simulink model "MPPT_vcte_temp"  (Simulink 7.4)
settings: Solver=ode3  StartTime=0.0  StopTime=6  FixedStep=1e-3  RelTol=1e-3
InitFcn:
  | % Ponto de linearização
  | D = 0.5;
  | L = 0.1;
  | C = 0.01;
  | R = 10;
  | Vo = 24;
  | Leq = L/(1-D)^2;
  | N = 1/(1-D);
libraries: simulink x4, powerlib_extras x1
settings Model: Creator=Luigi2  LastModifiedBy=Batlab
settings OptimizationCC: InitFltsAndDblsToZero=on
settings DebuggingCC: SaveWithParameterizedLinksMsg=none
settings GRTTargetCC: TargetFcnLib=ansi_tfl_tmw.mat

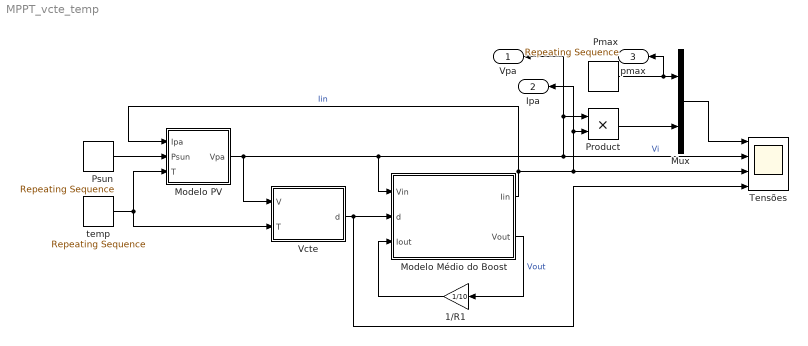
== system MPPT_vcte_temp ==
  1/R1 : Gain  Gain=1/10  ParameterDataType=sfix(16)  ParameterScaling=2^0  OutDataType=sfix(16)  OutScaling=2^0
  Modelo Médio do Boost : Subsystem  mask(Modelo de Pequenos Sinais do Boost){L=0.1, Iini=0, C=0.01, Vini=24}
      mask prompts: L "Indutância"; Iini "Corrente inicial"; C "Capacitância"; Vini "Tensão inicial"
      mask help:
      | São entradas do bloco:
      | Vin: Tensão de entrada
      | Iout: Corrente de saída
      | d: ciclo de trabalho
      |
      | São saídas do bloco:
      | Vout: Tensão de saída
      | Iin: Corrente de entrada
      |
      | Devem ser especificados a indutância, a capacitância e os seus valores iniciais para a utilização do modelo.
  Modelo PV : Subsystem
  Mux : Mux  Inputs=2
  Pmax : simulink/Sources/Repeating Sequence  SystemSampleTime=-1  rep_seq_t=[0 2 2 4 4 6]  rep_seq_y=[98.6721 98.6721 187.4175 187.4175 98.6721 98.6721]
  Product : Product  OutDataType=sfix(16)  OutScaling=2^0  RndMeth=Zero
  Psun : simulink/Sources/Repeating Sequence  SystemSampleTime=-1  rep_seq_t=[0 2 2 4 4 6]  rep_seq_y=[500 500 1000 1000 500 500]
  Tensões : Scope  NumInputPorts=4
      settings: TimeRange=6  YMin=-50~0~-2~0  YMax=250~40~10~0.4
  Vcte : Subsystem
  temp : simulink/Sources/Repeating Sequence  SystemSampleTime=-1  rep_seq_t=[0 2 2 4 4 6]  rep_seq_y=[25 25 40 40 25 25]
  Vpa : Outport  OutDataType=sfix(16)  OutScaling=2^0
  Ipa : Outport  Port=2  OutDataType=sfix(16)  OutScaling=2^0
  pmax : Outport  Port=3  OutDataType=sfix(16)  OutScaling=2^0
  wires:
  Modelo PV/1(Vpa) -> Tensões/2, Product/1, Vpa/1, Modelo Médio do Boost/1(Vin), Vcte/1(V)  "Vi"
  Modelo Médio do Boost/2(Vout) -> 1/R1/1  "Vout"
  1/R1/1 -> Modelo Médio do Boost/3(Iout)
  Modelo Médio do Boost/1(Iin) -> Tensões/3, Product/2, Ipa/1, Modelo PV/1(Ipa)  "Iin"
  Vcte/1(d) -> Tensões/4, Modelo Médio do Boost/2(d)
  Product/1 -> Mux/2
  Psun/1 -> Modelo PV/2(Psun)
  Pmax/1 -> Mux/1, pmax/1
  Mux/1 -> Tensões/1
  temp/1 -> Modelo PV/3(T), Vcte/2(T)

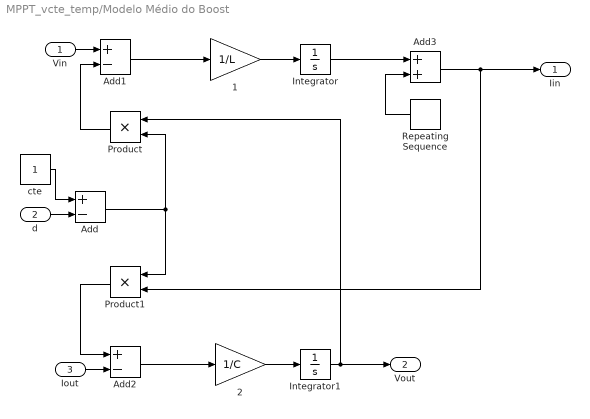
== system MPPT_vcte_temp/Modelo Médio do Boost ==
  Vin : Inport  OutDataType=sfix(16)  OutScaling=2^0
  d : Inport  Port=2  OutDataType=sfix(16)  OutScaling=2^0
  Iout : Inport  Port=3  OutDataType=sfix(16)  OutScaling=2^0
  1 : Gain  Gain=1/L  ParameterDataType=sfix(16)  ParameterScaling=2^0  OutDataType=sfix(16)  OutScaling=2^0
  2 : Gain  Gain=1/C  ParameterDataType=sfix(16)  ParameterScaling=2^0  OutDataType=sfix(16)  OutScaling=2^0
  Add : Sum  Inputs=+-  OutDataType=sfix(16)  OutScaling=2^-10
  Add1 : Sum  Inputs=+-  OutDataType=sfix(16)  OutScaling=2^-10
  Add2 : Sum  Inputs=+-  OutDataType=sfix(16)  OutScaling=2^-10
  Add3 : Sum  OutDataType=sfix(16)  OutScaling=2^-10
  Integrator : Integrator  InitialCondition=Iini
  Integrator1 : Integrator  InitialCondition=Vini
  Product : Product  OutDataType=sfix(16)  OutScaling=2^0  RndMeth=Zero
  Product1 : Product  OutDataType=sfix(16)  OutScaling=2^0  RndMeth=Zero
  Repeating Sequence : simulink/Sources/Repeating Sequence  SystemSampleTime=-1  rep_seq_t=[0 0.5/100 1/100]  rep_seq_y=[-1 1 -1]
  cte : Constant  OutDataType=sfix(16)  OutScaling=2^0
  Iin : Outport  OutDataType=sfix(16)  OutScaling=2^0
  Vout : Outport  Port=2  OutDataType=sfix(16)  OutScaling=2^0
  wires:
  Iout/1 -> Add2/2
  d/1 -> Add/2
  Vin/1 -> Add1/1
  Integrator1/1 -> Product/1, Vout/1
  2/1 -> Integrator1/1
  1/1 -> Integrator/1
  Add2/1 -> 2/1
  Product1/1 -> Add2/1
  Add1/1 -> 1/1
  Add/1 -> Product1/1, Product/2
  Product/1 -> Add1/2
  cte/1 -> Add/1
  Integrator/1 -> Add3/1
  Repeating Sequence/1 -> Add3/2
  Add3/1 -> Product1/2, Iin/1

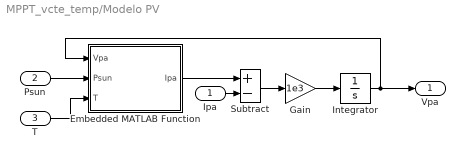
== system MPPT_vcte_temp/Modelo PV ==
  Ipa : Inport  OutDataType=sfix(16)  OutScaling=2^0
  Psun : Inport  Port=2  OutDataType=sfix(16)  OutScaling=2^0
  T : Inport  Port=3  OutDataType=sfix(16)  OutScaling=2^0
  Embedded MATLAB Function : Stateflow chart
  Gain : Gain  Gain=1e3  ParameterDataType=sfix(16)  ParameterScaling=2^0  OutDataType=sfix(16)  OutScaling=2^0
  Integrator : Integrator  LimitOutput=on  LowerSaturationLimit=0
  Subtract : Sum  Inputs=+-  OutDataType=sfix(16)  OutScaling=2^-10
  Vpa : Outport  OutDataType=sfix(16)  OutScaling=2^0
  wires:
  Psun/1 -> Embedded MATLAB Function/2(Psun)
  T/1 -> Embedded MATLAB Function/3(T)
  Embedded MATLAB Function/1(Ipa) -> Subtract/1
  Subtract/1 -> Gain/1
  Integrator/1 -> Embedded MATLAB Function/1(Vpa), Vpa/1
  Ipa/1 -> Subtract/2
  Gain/1 -> Integrator/1

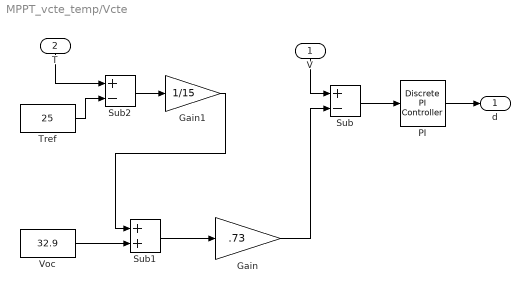
== system MPPT_vcte_temp/Vcte ==
  V : Inport  OutDataType=sfix(16)  OutScaling=2^0
  T : Inport  Port=2  OutDataType=sfix(16)  OutScaling=2^0
  Gain : Gain  Gain=.73  ParameterDataType=fixdt(1, 16)  ParameterScaling=2^0  OutDataType=fixdt(1, 16)  OutScaling=2^0
  Gain1 : Gain  Gain=1/15  ParameterDataType=fixdt(1, 16)  ParameterScaling=2^0  OutDataType=fixdt(1, 16)  OutScaling=2^0
  PI : powerlib_extras/Discrete  Control Blocks/Discrete PI Controller  DialogController=POWERSYS.PowerSysDialog  SystemSampleTime=-1  Kp=0.005  Ki=0.08  Par_Limits=[0.9 0]  Init=0  Ts=1e-3
  Sub : Sum  Inputs=+-  OutDataType=sfix(16)  OutScaling=2^-10
  Sub1 : Sum  Inputs=2  OutDataType=sfix(16)  OutScaling=2^-10
  Sub2 : Sum  Inputs=+-  OutDataType=sfix(16)  OutScaling=2^-10
  Tref : Constant  Value=25  OutDataType=sfix(16)  OutScaling=2^0
  Voc : Constant  Value=32.9  OutDataType=sfix(16)  OutScaling=2^0
  d : Outport  OutDataType=sfix(16)  OutScaling=2^0
  wires:
  V/1 -> Sub/1
  Sub/1 -> PI/1
  PI/1 -> d/1
  Voc/1 -> Sub1/2
  Sub1/1 -> Gain/1
  Gain/1 -> Sub/2
  T/1 -> Sub2/1
  Tref/1 -> Sub2/2
  Sub2/1 -> Gain1/1
  Gain1/1 -> Sub1/1

== matlab function Modelo PV/Embedded MATLAB Function ==
  data: Vpa input double; Ipa output double; Psun input double; T input double
function Ipa = PV_Array(Vpa, Psun, T) 
Rs = 0.005; 
Rp = 7; 
Ms = 1; % Módulos em Série
Mp = 1; % Módulos em Paralelo
Ns = 54; % No. de células
Voc = 32.9/Ns;
Isc = 8.21; 
a = 3.18e-3; 
n = 1.2; 
k = 1.38e-23; 
q = 1.60e-19; 
EG = 1.1; 
Tr = 273 + 25; 
T = 273 + T; 
Vt = n*k*T/q; 
V = Vpa/Ns/Ms; 
Iph = (Isc+a*(T-Tr))*Psun/1000; 
Irr = (Isc-Voc/Rp)/(exp(q*Voc/n/k/Tr)-1); 
Ir = Irr*(T/Tr)^3*exp(q*EG/n/k*(1/Tr-1/T)); 
I = 0; 
for j=1:5; 
I = I-(Iph-I-Ir*(exp((V+I*Rs)/Vt)-1)-(V+I*Rs)/Rp)/...
    (-1-Ir*exp((V+I*Rs)/Vt)*Rs/Vt-Rs/Rp); 
end 
if I<0, I=0; 
end 
Ipa = I*Mp;
